simulink model "Self_Excited_Induction_Motor"  (R2013b)
settings: Solver=ode23tb  SolverMode=SingleTasking  StartTime=0.0  StopTime=30  RelTol=1e-3
libraries: powerlib x20, powerlib_extras x1
Description:
  | Copyright 2008-2011 The MathWorks, Inc.
settings Model: ExtModeTrigMode=oneshot  ExtModeArmWhenConnect=off  ExtModeAutoUpdateStatusClock=off  Creator=MathWorks  LastModifiedBy=pc
settings DataIOCC: ExternalInput=[]  LimitDataPoints=off  SignalLoggingSaveFormat=ModelDataLogs  SaveOutput=off  SignalLogging=off  TimeSaveName=t  SignalLoggingName=sigsOut
settings OptimizationCC: BlockReduction=off  BooleanDataType=off  ExpressionDepthLimit=2147483647  InitFltsAndDblsToZero=on  EfficientMapNaN2IntZero=off
settings DebuggingCC: CheckExecutionContextPreStartOutputMsg=on  CheckExecutionContextRuntimeOutputMsg=on  SignalResolutionControl=TryResolveAllWithWarning  SolverPrmCheckMsg=none  MultiTaskDSMMsg=warning  MultiTaskCondExecSysMsg=none  SigSpecEnsureSampleTimeMsg=none  FcnCallInpInsideContextMsg=UseLocalSettings  UnconnectedInputMsg=none  UnconnectedOutputMsg=none  StateNameClashWarn=warning
settings HardwareCC: TargetUnknown=on
settings RTWCC: IncludeERTFirstTime=on
settings GRTTargetCC: CombineOutputUpdateFcns=off  GRTInterface=on

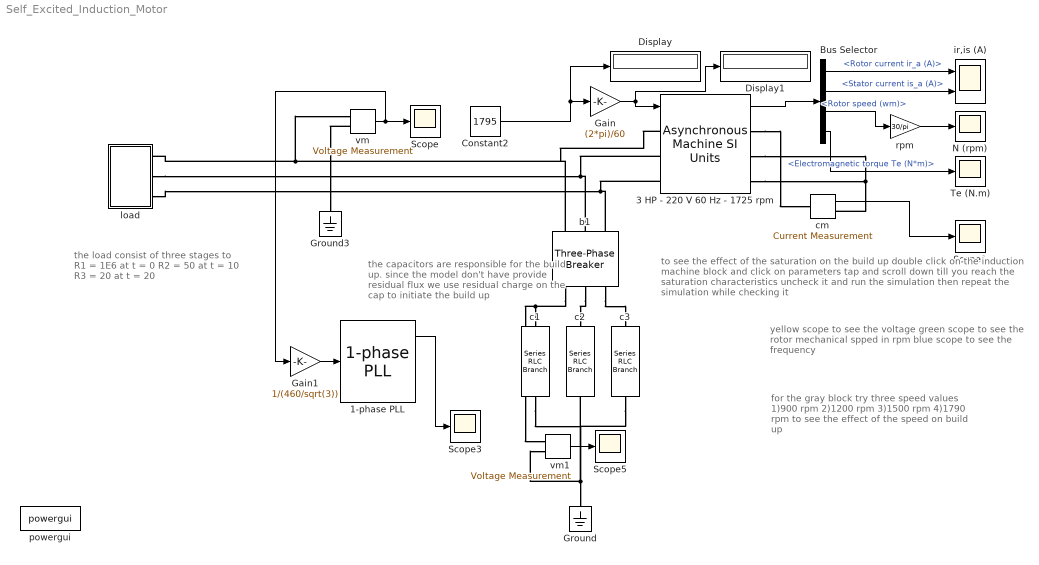
== system Self_Excited_Induction_Motor ==
  note: for the gray block try three speed values
      | 1)900 rpm
      | 2)1200 rpm
      | 3)1500 rpm
      | 4)1790 rpm
      | to see the effect of the speed on build up
  note: to see the effect of the saturation on the build up
      | double click on the induction machine block
      | and click on parameters tap and scroll down till you reach
      | the saturation characteristics
      | uncheck it and run the simulation then repeat the simulation while checking it
  note: the capacitors are responsible for
      | the build up. since the model don't
      | have provide residual flux we use residual
      | charge on the cap to initiate the build up
  note: the load consist of three stages to
      | R1 = 1E6 at t = 0
      | R2 = 50   at t = 10
      | R3 = 20   at t = 20
  note: yellow scope to see the voltage
      | green scope to see the rotor mechanical spped in rpm
      | blue scope to see the frequency
  1-phase PLL : powerlib_extras/Control  Blocks/1-phase PLL  Par_Init=[0 60]  ParK=[ 180 3200 1 ]  AGC=on
  3 HP - 220 V 60 Hz - 1725 rpm : powerlib/Machines/Asynchronous Machine SI Units  PresetModel=No  MechanicalLoad=Speed w  ShowDetailedParameters=on  RotorType=Wound  ReferenceFrame=Synchronous  NominalParameters=[3730 460 60]  Stator=[1.115 0.005974]  Rotor=[1.083 0.005974]  Cage1=[ 0.022 0.226/377]  Cage2=[ 0.022 0.226/377]  Lm=0.2037  Mechanical=[0.02 0.005752 2]  PolePairs=2  InitialConditions="[ 0.3,0   0,0,0   0,0,0 ]"  Units=SI  LoadFlowParameters=0  SimulateSaturation=on  Saturation=[1.403593122, 2.781365428, 5.379336849, 7.268890987, 9.798006896, 14.86815601, 21.57428561, 30.29841135, 42 ; 230, 322, 414, 460, 506, 552, 598, 644, 690]  TsPowergui=0  TsBlock=-1  IterativeModel=Forward Euler  Pmec=0
  Bus Selector : BusSelector  OutputSignals=Rotor measurements.Rotor current ir_a (A),Stator measurements.Stator current is_a (A),Mechanical.Rotor speed (wm),Mechanical.Electromagnetic torque Te (N*m)
  Constant2 : Constant  Value=1795
  Display : Display
  Display1 : Display
  Gain : Gain  Gain=(2*pi)/60
  Gain1 : Gain  Gain=1/(460/sqrt(3))
  Ground : powerlib/Elements/Ground  LConnTagsString=a
  Ground3 : powerlib/Elements/Ground  LConnTagsString=a
  N (rpm) : Scope
      settings: TimeRange=1  YMin=-200  YMax=1800  DataFormat=Structure
  Scope{,1,3,5} (4 alike) : Scope
      Scope settings: YMin=-55.25  YMax=-52.25
      Scope1 settings: SaveName=ScopeData2
      Scope3 settings: YMin=-100  YMax=90  SaveName=ScopeData3
      Scope5 settings: YMin=-1.125e-013  YMax=-8.75e-014  SaveName=ScopeData6
  Te (N.m) : Scope
      settings: YMin=-30  YMax=100  DataFormat=Structure
  b1 : powerlib/Elements/Three-Phase Breaker  InitialState=closed  SwitchA=off  SwitchB=off  SwitchC=off  SwitchTimes=[1]  External=off  BreakerResistance=0.000001  SnubberResistance=1e9  SnubberCapacitance=inf  Measurements=None
  c1 : powerlib/Elements/Series RLC Branch  LConnTagsString=__new0  RConnTagsString=__new0  BranchType=C  Resistance=1  Inductance=1e-3  SetiL0=off  InitialCurrent=0  Capacitance=1e-4  Setx0=on  InitialVoltage=0  Measurements=None
  c2 : powerlib/Elements/Series RLC Branch  LConnTagsString=__new0  RConnTagsString=__new0  BranchType=C  Resistance=1  Inductance=1e-3  SetiL0=off  InitialCurrent=0  Capacitance=1e-4  Setx0=on  InitialVoltage=sin(-120)  Measurements=None
  c3 : powerlib/Elements/Series RLC Branch  LConnTagsString=__new0  RConnTagsString=__new0  BranchType=C  Resistance=1  Inductance=1e-3  SetiL0=off  InitialCurrent=0  Capacitance=1e-4  Setx0=on  InitialVoltage=sin(120)  Measurements=None
  cm : powerlib/Measurements/Current Measurement  PhasorSimulation=off  OutputType=Complex  PSBequivalent=0
  ir,is (A) : Scope  NumInputPorts=2
      settings: YMin=-90~-90  YMax=90~90  DataFormat=Structure
  load : Subsystem
  powergui : powerlib/powergui  SimulationMode=Continuous  SolverType=Tustin  SampleTime=0  frequency=60  SPID=off  DisableSnubberDevices=off  DisableRonSwitches=off  DisableVfSwitches=off  SwTol=0  Interpol=off  DisplayEquations=off  frequencyindice=60  Pbase=100e6  ErrMax=1e-4  Iterations=50  UnitsV=kV  UnitsW=MW  FunctionMessages=off  echomessages=off  HookPort=off  EnableUseOfTLC=off  x0status=blocks  RestoreLinks=warning  ResistiveCurrentMeasurement=off  Frange=[0:2:500]  Ylog=off  Xlog=on  ShowGrid=off  save=off  variable=ZData  ZoomFFT=on  StartTime=0.0  cycles=1  DisplayStyle=1  fundamental=60  FreqAxis=off  MaxFrequency=1000  frequencyindicesteady=1  RmsSteady=1  display=off  Ts=0  methode=off
  rpm : Gain  Gain=30/pi  SaturateOnIntegerOverflow=on  OutDataTypeStr=Inherit: Same as input  ParamDataTypeStr=Inherit: Same as input
  vm : powerlib/Measurements/Voltage Measurement  PhasorSimulation=off  OutputType=Complex  PSBequivalent=0
  vm1 : powerlib/Measurements/Voltage Measurement  PhasorSimulation=off  OutputType=Complex  PSBequivalent=0
  wires:
  Bus Selector/4 -> Te (N.m)/1  "<Electromagnetic torque Te (N*m)>"
  rpm/1 -> N (rpm)/1
  Gain/1 -> 3 HP - 220 V 60 Hz - 1725 rpm/1, Display1/1
  Bus Selector/1 -> ir,is (A)/1  "<Rotor current ir_a (A)>"
  3 HP - 220 V 60 Hz - 1725 rpm/1 -> Bus Selector/1
  Bus Selector/2 -> ir,is (A)/2  "<Stator current is_a (A)>"
  Bus Selector/3 -> rpm/1  "<Rotor speed (wm)>"
  vm/1 -> Scope/1, Gain1/1
  cm/1 -> Scope1/1
  Constant2/1 -> Gain/1, Display/1
  vm1/1 -> Scope5/1
  1-phase PLL/1 -> Scope3/1
  Gain1/1 -> 1-phase PLL/1
  connections:
  b1/RConn1 -- c1/LConn1 -- vm1/LConn1
  b1/RConn2 -- c2/LConn1
  b1/RConn3 -- c3/LConn1
  c2/RConn1 -- c1/RConn1 -- c3/RConn1 -- Ground/LConn1 -- vm1/LConn2
  3 HP - 220 V 60 Hz - 1725 rpm/RConn1 -- cm/LConn1
  3 HP - 220 V 60 Hz - 1725 rpm/RConn2 -- cm/RConn1 -- 3 HP - 220 V 60 Hz - 1725 rpm/RConn3
  vm/LConn2 -- Ground3/LConn1
  3 HP - 220 V 60 Hz - 1725 rpm/LConn1 -- b1/LConn1 -- vm/LConn1 -- load/LConn1
  load/LConn2 -- 3 HP - 220 V 60 Hz - 1725 rpm/LConn2 -- b1/LConn2
  load/LConn3 -- 3 HP - 220 V 60 Hz - 1725 rpm/LConn3 -- b1/LConn3

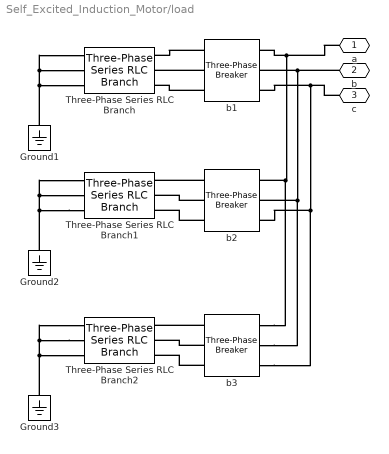
== system Self_Excited_Induction_Motor/load ==
  Ground1 : powerlib/Elements/Ground  LConnTagsString=a
  Ground2 : powerlib/Elements/Ground  LConnTagsString=a
  Ground3 : powerlib/Elements/Ground  LConnTagsString=a
  Three-Phase Series RLC Branch : powerlib/Elements/Three-Phase Series RLC Branch  LConnTagsString=A|B|C  RConnTagsString=A|B|C  BranchType=RL  Resistance=1e6  Inductance=1e-4  Capacitance=1e-6  Measurements=None
  Three-Phase Series RLC Branch1 : powerlib/Elements/Three-Phase Series RLC Branch  LConnTagsString=A|B|C  RConnTagsString=A|B|C  BranchType=RL  Resistance=50  Inductance=1e-4  Capacitance=1e-6  Measurements=None
  Three-Phase Series RLC Branch2 : powerlib/Elements/Three-Phase Series RLC Branch  LConnTagsString=A|B|C  RConnTagsString=A|B|C  BranchType=RL  Resistance=20  Inductance=1e-4  Capacitance=1e-6  Measurements=None
  b1 : powerlib/Elements/Three-Phase Breaker  InitialState=closed  SwitchA=off  SwitchB=off  SwitchC=off  SwitchTimes="[4/60  10/60]"  External=off  BreakerResistance=0.00001  SnubberResistance=1e9  SnubberCapacitance=inf  Measurements=None
  b2 : powerlib/Elements/Three-Phase Breaker  InitialState=open  SwitchA=on  SwitchB=on  SwitchC=on  SwitchTimes=[10]  External=off  BreakerResistance=0.00001  SnubberResistance=1e9  SnubberCapacitance=inf  Measurements=None
  b3 : powerlib/Elements/Three-Phase Breaker  InitialState=open  SwitchA=on  SwitchB=on  SwitchC=on  SwitchTimes=[20]  External=off  BreakerResistance=0.00001  SnubberResistance=1e9  SnubberCapacitance=inf  Measurements=None
  a : PMIOPort  Port=1  Side=Left
  b : PMIOPort  Port=2  Side=Left
  c : PMIOPort  Port=3  Side=Left
  connections:
  Ground1/LConn1 -- Three-Phase Series RLC Branch/LConn1 -- Three-Phase Series RLC Branch/LConn2 -- Three-Phase Series RLC Branch/LConn3
  b1/LConn1 -- Three-Phase Series RLC Branch/RConn1
  b1/LConn2 -- Three-Phase Series RLC Branch/RConn2
  b1/LConn3 -- Three-Phase Series RLC Branch/RConn3
  a/RConn1 -- b1/RConn1 -- b3/RConn1 -- b2/RConn1
  b/RConn1 -- b1/RConn2 -- b3/RConn2 -- b2/RConn2
  c/RConn1 -- b1/RConn3 -- b3/RConn3 -- b2/RConn3
  Three-Phase Series RLC Branch1/LConn3 -- Ground2/LConn1 -- Three-Phase Series RLC Branch1/LConn1 -- Three-Phase Series RLC Branch1/LConn2
  b2/LConn3 -- Three-Phase Series RLC Branch1/RConn3
  b2/LConn2 -- Three-Phase Series RLC Branch1/RConn2
  b2/LConn1 -- Three-Phase Series RLC Branch1/RConn1
  Three-Phase Series RLC Branch2/LConn2 -- Three-Phase Series RLC Branch2/LConn1 -- Three-Phase Series RLC Branch2/LConn3 -- Ground3/LConn1
  b3/LConn2 -- Three-Phase Series RLC Branch2/RConn2
  b3/LConn3 -- Three-Phase Series RLC Branch2/RConn3
  b3/LConn1 -- Three-Phase Series RLC Branch2/RConn1
